simulink model "sampleModel2072"  (R2023a)
settings: Solver=VariableStepAuto  StartTime=0.0  StopTime=10.0  RelTol=1e-3
libraries: hdlsllib x2, simulink x2
settings Model: Creator=user1  LastModifiedBy=user1

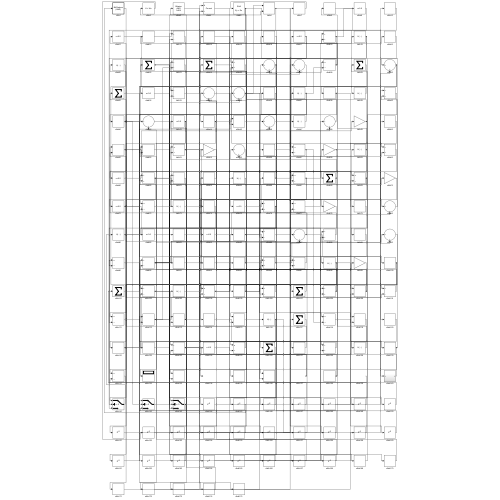
[thumbnail: Simulink's stored preview of the top-level diagram]
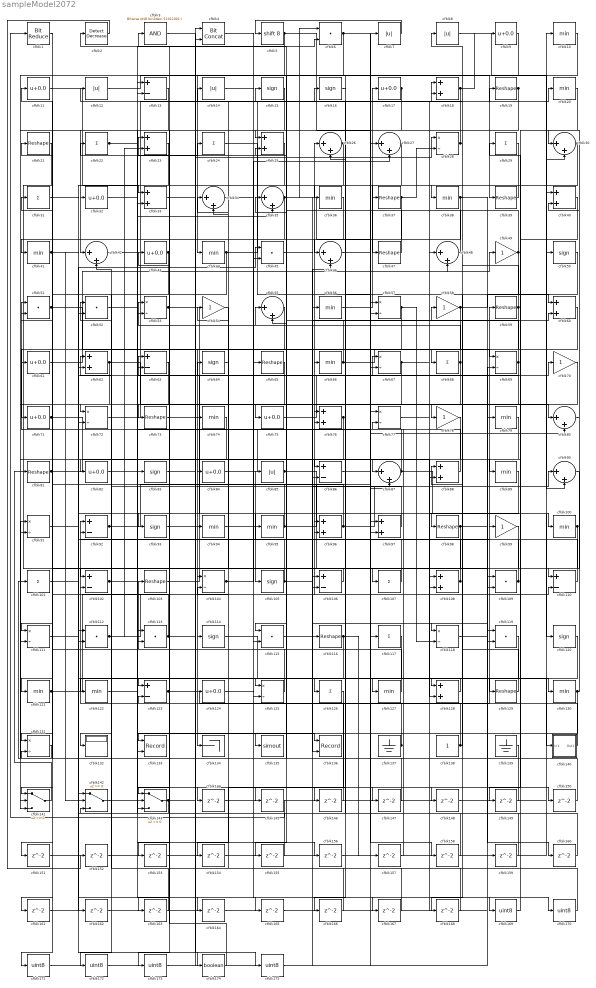
== system sampleModel2072 ==
  cfblk1 : hdlsllib/Logic and Bit Operations/Bit Reduce  mode=AND
  cfblk{10,20,36,38,41,44,56,66,74,79,89,94..95,100,121..122,127,130} (18 alike) : MinMax
  cfblk{22,24,29,31,68,101,107,117,126} (9 alike) : Sum  Inputs=+
  cfblk{13,63,86,92,102,106,110,123} (8 alike) : Sum  Inputs=+-
  cfblk{19,21,37,39,47,59,65,73,81,98,103,116,129} (13 alike) : Reshape
  cfblk{28,53,57,67,69,72,77,91,104,111,118,125,131} (13 alike) : Product  Inputs=*/  RndMeth=Zero  SaturateOnIntegerOverflow=on
  cfblk{15..16,50,64,83,93,105,114,120} (9 alike) : Signum
  cfblk{18,23,25,33,40,60,62,76,88,96..97,108,128} (13 alike) : Sum
  cfblk{6,45,51..52,109,112..113,115,119} (9 alike) : DotProduct  OutDataTypeStr=Inherit: Inherit via internal rule
  cfblk{9,11,17,32,43,61,71,75,82,84,124} (11 alike) : Bias  Bias=0.0  SaturateOnIntegerOverflow=off
  cfblk{7..8,12,14,85} (5 alike) : Abs  SaturateOnIntegerOverflow=off
  cfblk132 : Display
  cfblk133 : Record  FileSettingsInternal="{\"entries\":[{\"content\":{\"excelSettings\":{\"content\":{},\"type\":\"Streamout.ExcelSettings\"}},\"type\":\"Streamout.FileSettingStorage\",\"uuid\":\"\"}],\"packageUris\":[\"http:\\/\\/schema.mathworks.com\\/mf0\\/streamout_blocks\\/R2020a\"],\"version\":\"1.0\"}"  Layout=[1 1]  SignalsInternal="{\"entries\":[{\"content\":{\"signals\":[{\"content\":{\"blockPath\":[],\"dimensions\":[1],\"domain\":\"\",\"lineColor\":\"#a2142f\",\"plots\":[1],\"port\":1,\"signalID\":6494,\"signalName\":\"XY Graph:1\"},\"type\":\"RecordBlkView.Signal\",\"uuid\":\"\"},{\"content\":{\"blockPath\":[],\"dimensions\":[1],\"domain\":\"\",\"lineColor\":\"#139fff\",\"plots\":[1],\"port\":2,\"signalID\":6497,\"signalName\":\"XY Graph:2\"},\"type\":\"RecordBlkView.Signal\",\"uuid\":\"\"}]},\"type\":\"RecordBlkView.InputSignals\",\"uuid\":\"\"}],\"packageUris\":[\"http:\\/\\/schema.mathworks.com\\/mf0\\/streamout_blocks\\/R2020a\"],\"version\":\"1.0\"}"  VisualizationBindings="{\"xyplotplugin\":{\"info\":[{\"series\":[{\"bindingParametersList\":[{\"parameter\":\"X-Axis\",\"signalID\":6494,\"signalName\":\"XY Graph:1\"},{\"parameter\":\"Y-Axis\",\"signalID\":6497,\"signalName\":\"XY Graph:2\"}],\"seriesID\":26703}],\"subplotID\":1}]}}"  CompatibilityTag=XY  st=-1
  cfblk134 : Terminator
  cfblk135 : ToWorkspace  VariableName=simout  SaveFormat=Timeseries  SampleTime=-1
  cfblk136 : Record  FileSettingsInternal="{\"entries\":[{\"content\":{\"excelSettings\":{\"content\":{},\"type\":\"Streamout.ExcelSettings\"}},\"type\":\"Streamout.FileSettingStorage\",\"uuid\":\"\"}],\"packageUris\":[\"http:\\/\\/schema.mathworks.com\\/mf0\\/streamout_blocks\\/R2020a\"],\"version\":\"1.0\"}"  Layout=[1 1]  SignalsInternal="{\"entries\":[{\"content\":{\"signals\":[{\"content\":{\"blockPath\":[],\"dimensions\":[1],\"domain\":\"\",\"lineColor\":\"#a2142f\",\"plots\":[1],\"port\":1,\"signalID\":6502,\"signalName\":\"XY Graph:1\"},\"type\":\"RecordBlkView.Signal\",\"uuid\":\"\"},{\"content\":{\"blockPath\":[],\"dimensions\":[1],\"domain\":\"\",\"lineColor\":\"#139fff\",\"plots\":[1],\"port\":2,\"signalID\":6505,\"signalName\":\"XY Graph:2\"},\"type\":\"RecordBlkView.Signal\",\"uuid\":\"\"}]},\"type\":\"RecordBlkView.InputSignals\",\"uuid\":\"\"}],\"packageUris\":[\"http:\\/\\/schema.mathworks.com\\/mf0\\/streamout_blocks\\/R2020a\"],\"version\":\"1.0\"}"  VisualizationBindings="{\"xyplotplugin\":{\"info\":[{\"series\":[{\"bindingParametersList\":[{\"parameter\":\"X-Axis\",\"signalID\":6502,\"signalName\":\"XY Graph:1\"},{\"parameter\":\"Y-Axis\",\"signalID\":6505,\"signalName\":\"XY Graph:2\"}],\"seriesID\":43252}],\"subplotID\":1}]}}"  CompatibilityTag=XY  st=-1
  cfblk137 : Ground
  cfblk138 : Constant  SampleTime=-1
  cfblk139 : Ground
  cfblk140 : Subsystem
      settings: LibrarySourceBlock=|
      | hdlsllib/Ports &
      | Subsystems/Subsystem
  cfblk141 : Switch  SaturateOnIntegerOverflow=off  InputSameDT=off
  cfblk142 : Switch  SaturateOnIntegerOverflow=off  InputSameDT=off
  cfblk143 : Switch  SaturateOnIntegerOverflow=off  InputSameDT=off
  cfblk{144..168} (25 alike) : Delay  SampleTime=1
  cfblk{169..173,175} (6 alike) : DataTypeConversion  OutDataTypeStr=uint8  SaturateOnIntegerOverflow=off  RndMeth=Floor
  cfblk174 : DataTypeConversion  OutDataTypeStr=boolean  SaturateOnIntegerOverflow=off  RndMeth=Floor
  cfblk2 : simulink/Logic and Bit Operations/Detect Decrease  vinit=0.0  OutDataTypeStr=boolean
      settings: LibrarySourceBlock=|
      | hdlsllib/Logic and Bit
      | Operations/Detect
      | Decrease
  cfblk{26..27,30,34..35,42,46,48,55,80,87,90} (12 alike) : Sum  Inputs=|++
  cfblk3 : simulink/Logic and Bit Operations/Bitwise Operator  logicop=AND  UseBitMask=on  BitMask=bin2dec('11011001')  BitMaskRealWorld=Stored Integer
      settings: LibrarySourceBlock=|
      | hdlsllib/Logic and Bit
      | Operations/Bitwise
      | Operator
  cfblk4 : hdlsllib/Logic and Bit Operations/Bit Concat  numInputs=2
  cfblk{49,54,58,70,78,99} (6 alike) : Gain
  cfblk5 : ArithShift  BitShiftNumber=8
  wires:
  cfblk17/1 -> cfblk42/1, cfblk57/2
  cfblk25/1 -> cfblk32/1
  cfblk61/1 -> cfblk48/2
  cfblk125/1 -> cfblk103/1
  cfblk123/1 -> cfblk59/1, cfblk76/2, cfblk148/1
  cfblk21/1 -> cfblk107/1
  cfblk81/1 -> cfblk87/1, cfblk45/1
  cfblk38/1 -> cfblk79/1, cfblk72/2
  cfblk137/1 -> cfblk92/1, cfblk104/2
  cfblk66/1 -> cfblk68/1, cfblk25/2
  cfblk112/1 -> cfblk26/1, cfblk23/2, cfblk76/1
  cfblk72/1 -> cfblk15/1
  cfblk12/1 -> cfblk39/1
  cfblk103/1 -> cfblk67/1
  cfblk116/1 -> cfblk122/1, cfblk155/1, cfblk157/1
  cfblk56/1 -> cfblk17/1
  cfblk39/1 -> cfblk33/1
  cfblk18/1 -> cfblk9/1, cfblk153/1
  cfblk65/1 -> cfblk75/1
  cfblk82/1 -> cfblk113/2
  cfblk94/1 -> cfblk105/1
  cfblk100/1 -> cfblk115/1, cfblk151/1
  cfblk88/1 -> cfblk51/1
  cfblk79/1 -> cfblk82/1
  cfblk93/1 -> cfblk66/1
  cfblk37/1 -> cfblk131/1, cfblk28/2, cfblk112/2
  cfblk67/1 -> cfblk134/1, cfblk91/2, cfblk60/2
  cfblk106/1 -> cfblk102/1
  cfblk104/1 -> cfblk99/1, cfblk27/2
  cfblk97/1 -> cfblk62/1
  cfblk49/1 -> cfblk23/1, cfblk166/1
  cfblk44/1 -> cfblk18/1, cfblk173/1
  cfblk30/1 -> cfblk47/1, cfblk36/1
  cfblk129/1 -> cfblk88/1
  cfblk80/1 -> cfblk30/1
  cfblk23/1 -> cfblk62/2
  cfblk51/1 -> cfblk109/1, cfblk143/3
  cfblk71/1 -> cfblk108/2, cfblk167/1
  cfblk7/1 -> cfblk5/1
  cfblk113/1 -> cfblk11/1, cfblk20/1
  cfblk73/1 -> cfblk78/1
  cfblk99/1 -> cfblk114/1
  cfblk53/1 -> cfblk98/1, cfblk127/1
  cfblk41/1 -> cfblk128/1, cfblk142/2, cfblk93/1
  cfblk131/1 -> cfblk101/1
  cfblk27/1 -> cfblk73/1
  cfblk29/1 -> cfblk38/1
  cfblk139/1 -> cfblk131/2
  cfblk143/1 -> cfblk124/1, cfblk142/3
  cfblk11/1 -> cfblk33/2
  cfblk6/1 -> cfblk44/1, cfblk158/1
  cfblk140/1(Out1) -> cfblk92/2
  cfblk20/1 -> cfblk129/1
  cfblk55/1 -> cfblk71/1
  cfblk102/1 -> cfblk24/1, cfblk35/2
  cfblk130/1 -> cfblk133/1, cfblk40/2
  cfblk62/1 -> cfblk80/1, cfblk6/2, cfblk111/1
  cfblk26/1 -> cfblk86/1, cfblk52/2
  cfblk96/1 -> cfblk50/1, cfblk21/1
  cfblk13/1 -> cfblk61/1
  cfblk19/1 -> cfblk55/2, cfblk111/2
  cfblk128/1 -> cfblk123/1
  cfblk98/1 -> cfblk130/1, cfblk141/1, cfblk161/1
  cfblk32/1 -> cfblk136/1
  cfblk10/1 -> cfblk125/1
  cfblk110/1 -> cfblk63/1
  cfblk16/1 -> cfblk46/1
  cfblk63/1 -> cfblk132/1
  cfblk34/1 -> cfblk125/2
  cfblk105/1 -> cfblk90/1, cfblk58/1, cfblk85/1
  cfblk42/1 -> cfblk100/1
  cfblk35/1 -> cfblk57/1, cfblk6/1, cfblk118/1, cfblk41/1
  cfblk74/1 -> cfblk133/2
  cfblk48/1 -> cfblk37/1
  cfblk77/1 -> cfblk19/1
  cfblk138/1 -> cfblk18/2, cfblk96/2
  cfblk60/1 -> cfblk84/1
  cfblk54/1 -> cfblk104/1
  cfblk101/1 -> cfblk70/1
  cfblk109/1 -> cfblk34/1, cfblk42/2
  cfblk8/1 -> cfblk90/2
  cfblk59/1 -> cfblk12/1, cfblk115/2
  cfblk57/1 -> cfblk97/2, cfblk118/2
  cfblk40/1 -> cfblk89/1
  cfblk75/1 -> cfblk7/1
  cfblk14/1 -> cfblk69/1
  cfblk68/1 -> cfblk53/1, cfblk74/1
  cfblk92/1 -> cfblk13/2, cfblk80/2, cfblk65/1, cfblk164/1, cfblk165/1
  cfblk141/1 -> cfblk81/1
  cfblk95/1 -> cfblk54/1, cfblk49/1
  cfblk24/1 -> cfblk77/1
  cfblk85/1 -> cfblk119/1, cfblk46/2
  cfblk127/1 -> cfblk31/1
  cfblk91/1 -> cfblk106/2
  cfblk64/1 -> cfblk14/1
  cfblk43/1 -> cfblk121/1, cfblk72/1
  cfblk121/1 -> cfblk10/1, cfblk96/1
  cfblk5/1 -> cfblk87/2, cfblk141/3, cfblk45/2
  cfblk9/1 -> cfblk126/1
  cfblk69/1 -> cfblk63/2, cfblk135/1, cfblk22/1
  cfblk45/1 -> cfblk56/1
  cfblk36/1 -> cfblk86/2
  cfblk28/1 -> cfblk25/1, cfblk8/1
  cfblk107/1 -> cfblk52/1
  cfblk90/1 -> cfblk110/1
  cfblk87/1 -> cfblk120/1, cfblk16/1
  cfblk47/1 -> cfblk2/1
  cfblk76/1 -> cfblk136/2, cfblk141/2
  cfblk52/1 -> cfblk83/1
  cfblk86/1 -> cfblk119/2
  cfblk58/1 -> cfblk143/1, cfblk60/1
  cfblk108/1 -> cfblk64/1, cfblk35/1
  cfblk142/1 -> cfblk53/2
  cfblk83/1 -> cfblk94/1
  cfblk84/1 -> cfblk27/1
  cfblk115/1 -> cfblk110/2
  cfblk89/1 -> cfblk128/2
  cfblk33/1 -> cfblk28/1
  cfblk15/1 -> cfblk143/2
  cfblk114/1 -> cfblk140/1(In1)
  cfblk22/1 -> cfblk95/1, cfblk144/1
  cfblk144/1 -> cfblk69/2
  cfblk70/1 -> cfblk145/1
  cfblk145/1 -> cfblk1/1
  cfblk119/1 -> cfblk146/1
  cfblk146/1 -> cfblk13/1
  cfblk124/1 -> cfblk147/1
  cfblk147/1 -> cfblk91/1
  cfblk148/1 -> cfblk40/1
  cfblk120/1 -> cfblk149/1
  cfblk149/1 -> cfblk55/1
  cfblk46/1 -> cfblk150/1
  cfblk150/1 -> cfblk51/2
  cfblk151/1 -> cfblk108/1
  cfblk2/1 -> cfblk152/1
  cfblk152/1 -> cfblk30/2
  cfblk153/1 -> cfblk67/2
  cfblk126/1 -> cfblk154/1
  cfblk155/1 -> cfblk113/1
  cfblk122/1 -> cfblk156/1
  cfblk156/1 -> cfblk97/1
  cfblk157/1 -> cfblk77/2
  cfblk158/1 -> cfblk26/2
  cfblk159/1 -> cfblk142/1
  cfblk118/1 -> cfblk160/1
  cfblk160/1 -> cfblk123/2
  cfblk161/1 -> cfblk112/1
  cfblk31/1 -> cfblk162/1
  cfblk162/1 -> cfblk48/1
  cfblk78/1 -> cfblk163/1
  cfblk163/1 -> cfblk102/2
  cfblk164/1 -> cfblk109/2
  cfblk165/1 -> cfblk88/2
  cfblk166/1 -> cfblk106/1
  cfblk167/1 -> cfblk34/2
  cfblk50/1 -> cfblk168/1
  cfblk168/1 -> cfblk43/1
  cfblk4/1 -> cfblk169/1
  cfblk169/1 -> cfblk29/1
  cfblk154/1 -> cfblk170/1
  cfblk170/1 -> cfblk4/1
  cfblk1/1 -> cfblk171/1
  cfblk171/1 -> cfblk4/2
  cfblk117/1 -> cfblk172/1
  cfblk172/1 -> cfblk116/1
  cfblk173/1 -> cfblk117/1
  cfblk111/1 -> cfblk174/1
  cfblk174/1 -> cfblk3/1
  cfblk3/1 -> cfblk175/1
  cfblk175/1 -> cfblk159/1

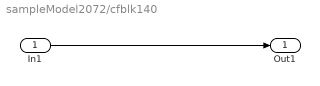
== system sampleModel2072/cfblk140 ==
  In1 : Inport
  Out1 : Outport
  wires:
  In1/1 -> Out1/1
